simulink model "controlledmotorposition"  (R2020b)
settings: Solver=VariableStepAuto  StartTime=0.0  StopTime=10.0  RelTol=1e-3
undefined symbols (not defined in the file): b, J, Kd, Ke, Ki, Kp, Kt, L, R
settings Model: Creator=HP  LastModifiedBy=HP

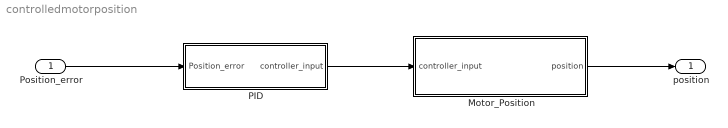
== system controlledmotorposition ==
  Position_error : Inport  OutDataTypeStr=double  PortDimensions=1  SampleTime=0
  Motor_Position : Subsystem
  PID : Subsystem
  position : Outport  OutDataTypeStr=double  PortDimensions=1  SampleTime=0
  wires:
  PID/1(controller_input) -> Motor_Position/1(controller_input)
  Position_error/1 -> PID/1(Position_error)
  Motor_Position/1(position) -> position/1

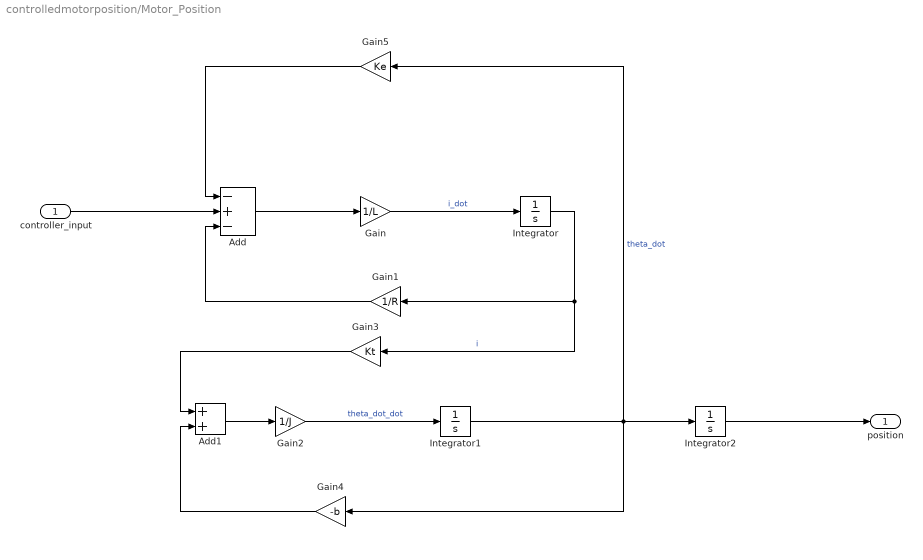
== system controlledmotorposition/Motor_Position ==
  controller_input : Inport
  Add : Sum  Inputs=-+-
  Add1 : Sum
  Gain : Gain  Gain=1/L
  Gain1 : Gain  Gain=1/R
  Gain2 : Gain  Gain=1/J
  Gain3 : Gain  Gain=Kt
  Gain4 : Gain  Gain=-b
  Gain5 : Gain  Gain=Ke
  Integrator : Integrator
  Integrator1 : Integrator
  Integrator2 : Integrator
  position : Outport
  wires:
  controller_input/1 -> Add/2
  Integrator2/1 -> position/1
  Gain5/1 -> Add/1
  Gain4/1 -> Add1/2
  Gain2/1 -> Integrator1/1  "theta_dot_dot"
  Gain1/1 -> Add/3
  Add/1 -> Gain/1
  Integrator1/1 -> Integrator2/1, Gain5/1, Gain4/1  "theta_dot"
  Add1/1 -> Gain2/1
  Integrator/1 -> Gain1/1, Gain3/1  "i"
  Gain/1 -> Integrator/1  "i_dot"
  Gain3/1 -> Add1/1

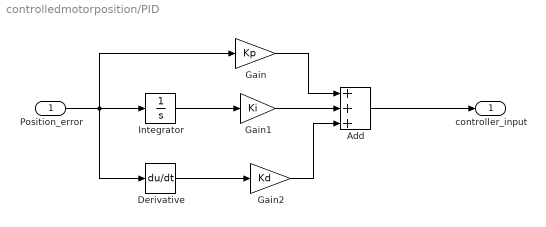
== system controlledmotorposition/PID ==
  Position_error : Inport
  Add : Sum  Inputs=+++
  Derivative : Derivative
  Gain : Gain  Gain=Kp
  Gain1 : Gain  Gain=Ki
  Gain2 : Gain  Gain=Kd
  Integrator : Integrator
  controller_input : Outport
  wires:
  Gain/1 -> Add/1
  Gain2/1 -> Add/3
  Position_error/1 -> Integrator/1, Derivative/1, Gain/1
  Add/1 -> controller_input/1
  Gain1/1 -> Add/2
  Integrator/1 -> Gain1/1
  Derivative/1 -> Gain2/1
